simulink model "Watermark_System"  (R2024b)
settings: Solver=VariableStepAuto  StartTime=0.0  StopTime=10.0  RelTol=1e-3
undefined symbols (not defined in the file): Cq, Cw, Dq, Dw, Gq, Gw, Hq, Hw, start_time, start_time_QW
settings Model: Creator=54238  LastModifiedBy=54238

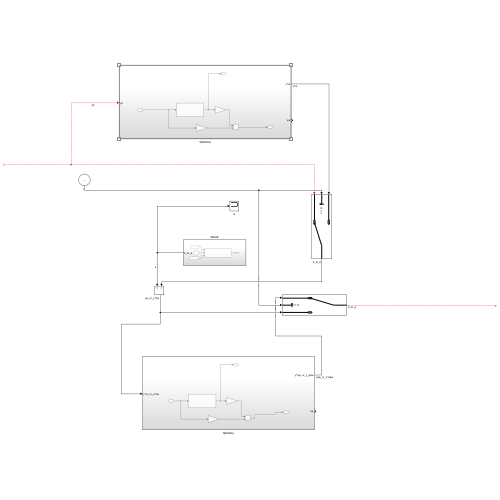
[thumbnail: Simulink's stored preview of the top-level diagram]
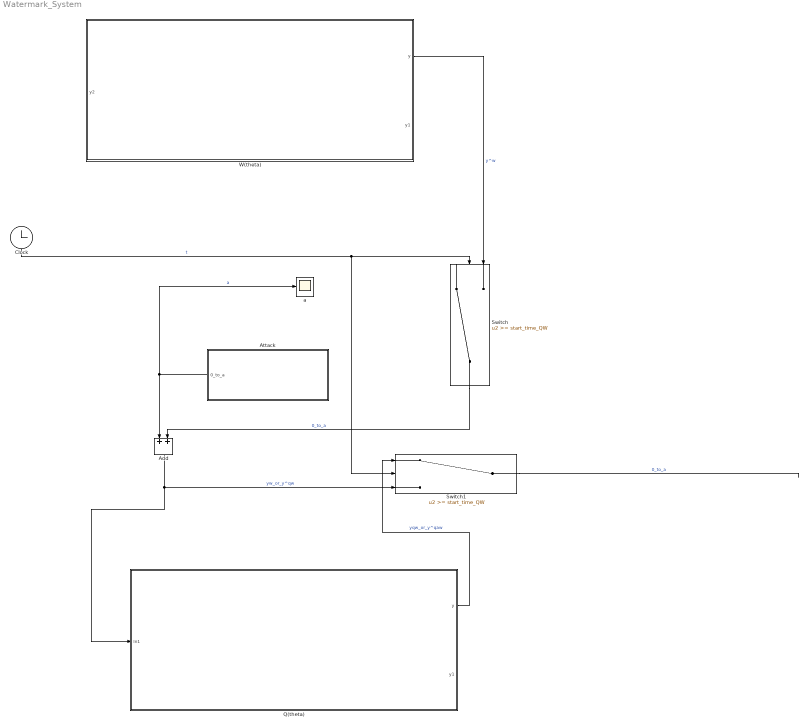
== system Watermark_System ==
  Add : Sum
  Attack : Subsystem
  Clock : Clock
  Q(theta) : Subsystem
  Switch : Switch  Threshold=start_time_QW  SaturateOnIntegerOverflow=off  InputSameDT=off
  Switch1 : Switch  Threshold=start_time_QW  SaturateOnIntegerOverflow=off  InputSameDT=off
  W(theta) : Subsystem
  a : Scope
  wires:
  ? -> Switch/1, W(theta)/1(y2)  "y0"
  W(theta)/1(y) -> Switch/3  "y^w"
  Switch1/1 -> ?  "0_to_a"
  Attack/1(0_to_a) -> Add/1, a/1  "a"
  Q(theta)/1(y) -> Switch1/1  "yqw_or_y^qaw"
  Add/1 -> Switch1/3, Q(theta)/1(In1)  "yw_or_y^qw"
  Clock/1 -> Switch1/2, Switch/2  "t"
  Switch/1 -> Add/2  "0_to_a"

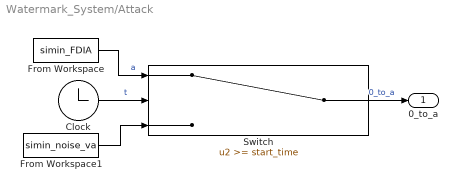
== system Watermark_System/Attack ==
  Clock : Clock
  From Workspace : FromWorkspace  VariableName=simin_FDIA  SampleTime=-1
  From Workspace1 : FromWorkspace  VariableName=simin_noise_va  SampleTime=-1
  Switch : Switch  Threshold=start_time  SaturateOnIntegerOverflow=off  InputSameDT=off
  0_to_a : Outport
  wires:
  From Workspace1/1 -> Switch/3
  Clock/1 -> Switch/2  "t"
  From Workspace/1 -> Switch/1  "a"
  Switch/1 -> 0_to_a/1  "0_to_a"

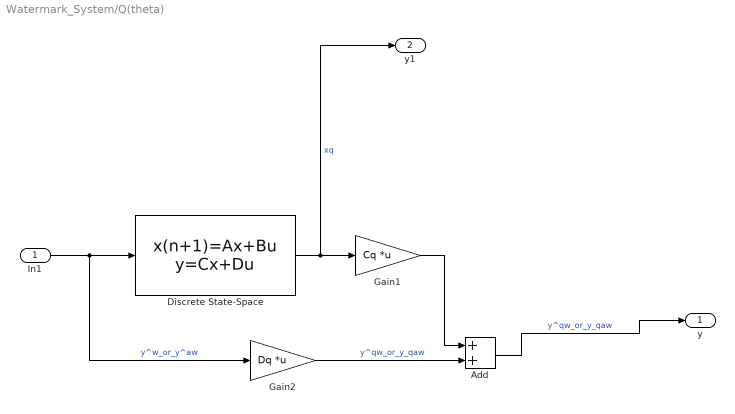
== system Watermark_System/Q(theta) ==
  In1 : Inport
  Add : Sum
  Discrete State-Space : DiscreteStateSpace  A=Gq  B=Hq  C=[1 0 0 0;0 1 0 0;0 0 1 0;0 0 0 1]  D=[0 0;0 0;0 0;0 0]  InitialCondition=[0 0 0 0]  SampleTime=-1
  Gain1 : Gain  Gain=Cq  Multiplication=Matrix(K*u)
  Gain2 : Gain  Gain=Dq  Multiplication=Matrix(K*u)
  y : Outport
  y1 : Outport  Port=2
  wires:
  Discrete State-Space/1 -> y1/1, Gain1/1  "xq"
  In1/1 -> Gain2/1, Discrete State-Space/1  "y^w_or_y^aw"
  Gain1/1 -> Add/1
  Gain2/1 -> Add/2  "y^qw_or_y_qaw"
  Add/1 -> y/1  "y^qw_or_y_qaw"

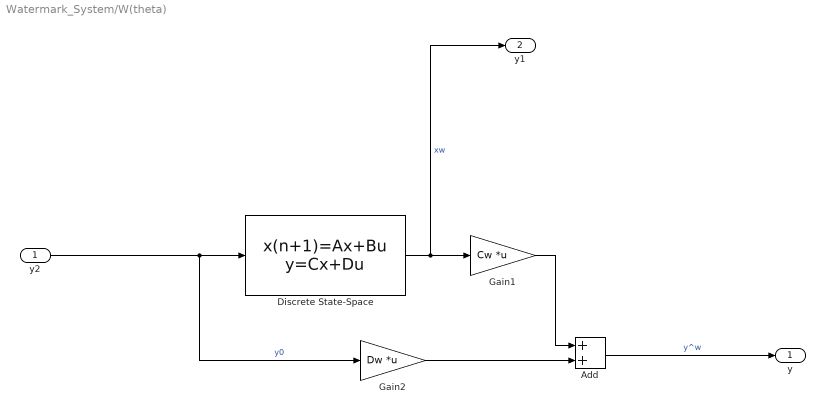
== system Watermark_System/W(theta) ==
  y2 : Inport
  Add : Sum
  Discrete State-Space : DiscreteStateSpace  A=Gw  B=Hw  C=[1 0 0 0;0 1 0 0;0 0 1 0;0 0 0 1]  D=[0 0;0 0;0 0;0 0]  InitialCondition=[0 0 0 0]  SampleTime=-1
  Gain1 : Gain  Gain=Cw  Multiplication=Matrix(K*u)
  Gain2 : Gain  Gain=Dw  Multiplication=Matrix(K*u)
  y : Outport
  y1 : Outport  Port=2
  wires:
  Discrete State-Space/1 -> y1/1, Gain1/1  "xw"
  y2/1 -> Gain2/1, Discrete State-Space/1  "y0"
  Gain1/1 -> Add/1
  Gain2/1 -> Add/2
  Add/1 -> y/1  "y^w"
